simulink model "pfc_simulation"  (R2025b)
settings: Solver=ode23t  StartTime=0.0  StopTime=3  FixedStep=15.625e-6  RelTol=1e-3  EnableMultiTasking=on
PostLoadFcn:
  | mchp_pfc_foc_dsPIC33A_data
values from neighbouring files (symbols this model uses):
  R = (Vout^2)/Po    (= 96.2666666667)    [mchp_pfc_foc_dsPIC33A_data.m]
  Ts = T_pwm    (= 1.5625e-05)    [mchp_pfc_foc_dsPIC33A_data.m]
undefined symbols (not defined in the file or in its folder): Down, f_sw, Up
libraries: ee_lib x8, fl_lib x7, nesl_utility x7, eeGeneralControl x1
settings Model: ExtModeEnableFloating=off  ExtModeTrigDuration=20  Creator=I50990  LastModifiedBy=Andy
settings SolverCC: AlgebraicLoopSolver=TrustRegion
settings OptimizationCC: DefaultParameterBehavior=Inlined  DefaultUnderspecifiedDataType=single  InlineInvariantSignals=on  EnhancedBackFolding=on  BooleansAsBitfields=on  PassReuseOutputArgsAs=Individual arguments  ZeroExternalMemoryAtStartup=off  ZeroInternalMemoryAtStartup=off  OptimizeBlockOrder=speed  DifferentSizesBufferReuse=on  EfficientTunableParamExpr=on
settings DebuggingCC: MultiTaskDSMMsg=none  MultiTaskCondExecSysMsg=none  MultiTaskRateTransMsg=warning  ParameterTunabilityLossMsg=error  ArithmeticOperatorsInVariantConditions=warning
settings HardwareCC: ProdBitPerPointer=32.0  ProdBitPerSizeT=32.0  ProdBitPerPtrDiffT=32.0  ProdLargestAtomicInteger=Long  ProdWordSize=32.0  ProdLongLongMode=on  ProdHWDeviceType=Generic->Custom
settings ModelReferenceCC: ModelReferenceNumInstancesAllowed=Single
settings SFSimCC: MATLABDynamicMemAlloc=off  CustomCodeUndefinedFunction=UseInterfaceOnly
settings RTWCC: SystemTargetFile=MCHP_dsPIC33A_stf.tlc  TLCOptions="-aExtModeXCPClassicInterface=0  -aCreateExtModeTypes=1 -aExtModeXCPSimulationTimeInTicks=1"  TemplateMakefile=MCHP_dsPIC33A.tmf  GPUComputeCapability=3.5  Description=Microchip Embedded Target dsPIC33A (real-time)
settings CodeAppCC: ForceParamTrailComments=on  IgnoreCustomStorageClasses=off  MaxIdLength=255.0  OperatorAnnotations=on  SimulinkDataObjDesc=on  SFDataObjDesc=on  InsertBlockDesc=on
settings STFCustomTargetCC: SystemTargetFile=MCHP_dsPIC33A_stf.tlc  TargetLibSuffix=_lib.a  TargetLangStandard=C99 (ISO)  MultiwordLength=256.0  ConcurrentExecutionCompliant=off  CombineOutputUpdateFcns=on  CombineSignalStateStructs=on  ERTCustomFileBanners=on  SupportContinuousTime=off  RemoveResetFunc=on  MATLABClassNameForMDSCustomization=Simulink.SoftwareTarget.ERTCustomization  GRTInterface=off  TIMER_PERIOD="[0  65535]"  GCC1=xc-dsc-gcc.exe  AR1=xc-dsc-ar  OPTIM_GCC=-O2 -mno-eds-warn -mconst-in-data -mlarge-code -mlarge-data -mlarge-scalar -mlarge-aggregate -g -Wa,--reorder  GCCPATH=C:/PROGRA~1/MICROC~1/xc-dsc/v3.21/bin  AssemblyListing=off  MCHP_XCP_MemoryBlockParameters=[-1 8]  LINKER_SCRIPT=p33AK128MC106.gld  ProduceHexOutput=off  HOST_PLATFORM=PC  BIN2HEX=xc-dsc-bin2hex  TIMER_START="[0  0]"  RTWGenSettings_txt="s.UART_TX_IMPLEMENTATION='[2  2]';s.UART_RX_IMPLEMENTATION='[2  2]';s.UART_TX_DMACHANNEL='[2  1]';s.UART_HALF_DUPLEX_MODE='[0  0]';s.UART_TX_THREAD_PROTECTION='[9  9]';s.RefMasterBlk='pfc_model_simulation/MCHV-230VAC-1.5kW Development Board dsPIC33AK128MC106 MC DIM/Microchip Master';s.ChipIdN='[33  128  106]';s.ChipIdL1='AK';s.ChipIdL2='MC';s.ChipIdL3='';s.arch3='33A';s.ChipId='33AK128MC106';s.Arch='8';s.bitFieldsSFR='3';s.ChipRAM='16384';s.ChipRAM_XBegin='16384';s.ChipRAM_dma='[-1 -1]';s.FuseConfigTxt='#pragma config FWDT_WDTEN = SW\\\\n#pragma config FICD_JTAGEN = OFF\\\\n';s.TimeStep_Timer='-1';s.TimeStep_SyncADC='1';s.ADPCFG='0';s.ANSEL_Exist='1';s.ANSEL='[-1 -1 -1 -1 -1 -1 -1 -1 -1 -1 -1]';s.TRIS='[65535  65535  64990  65503     -1     -1     -1     -1     -1     -1     -1     -1     -1     -1     -1     -1     -1     -1     -1     -1     -1     -1     -1     -1     -1     -1     -1     -1     -1     -1     -1     -1     -1     -1     -1     -1     -1     -1     -1     -1     -1     -1     -1     -1     -1     -1     -1     -1     -1     -1     -1     -1     -1     -1     -1     -1     -1]';s.RPOR='[-1         -1         -1         -1         -1         -1         -1         -1         -1         -1     589824         -1         -1         -1  184549376         -1         -1         -1         -1         -1]';s.RPINR='[-1       -1       -1       -1       -1       -1       -1       -1       -1  3997740       -1       -1       -1       -1       -1       -1       -1       -1       -1       -1       -1       -1]';s.LATSET='[-1 -1 -1 -1 -1 -1 -1 -1 -1 -1 -1 -1 -1 -1 -1 -1 -1 -1 -1 -1 -1 -1 -1 -1 -1 -1 -1 -1 -1 -1 -1 -1 -1 -1 -1 -1 -1 -1 -1 -1 -1 -1 -1 -1 -1 -1 -1 -1 -1 -1 -1 -1 -1 -1 -1 -1 -1]';s.LATCLR='[-1 -1 -1 -1 -1 -1 -1 -1 -1 -1 -1 -1 -1 -1 -1 -1 -1 -1 -1 -1 -1 -1 -1 -1 -1 -1 -1 -1 -1 -1 -1 -1 -1 -1 -1 -1 -1 -1 -1 -1 -1 -1 -1 -1 -1 -1 -1 -1 -1 -1 -1 -1 -1 -1 -1 -1 -1]';s.ODC='[-1 -1 -1 -1 -1 -1 -1 -1 -1 -1 -1 -1 -1 -1 -1 -1 -1 -1 -1 -1 -1 -1 -1 -1 -1 -1 -1 -1 -1 -1 -1 -1 -1 -1 -1 -1 -1 -1 -1 -1 -1 -1 -1 -1 -1 -1 -1 -1 -1 -1 -1 -1 -1 -1 -1 -1 -1]';s.CNPU='[-1 -1 -1 -1 -1 -1 -1 -1 -1 -1 -1 -1 -1 -1 -1 -1 -1 -1 -1 -1 -1 -1 -1 -1 -1 -1 -1 -1 -1 -1 -1 -1 -1 -1 -1 -1 -1 -1 -1 -1 -1 -1 -1 -1 -1 -1 -1 -1 -1 -1 -1 -1 -1 -1 -1 -1 -1]';s.CNPD='[-1 -1 -1 -1 -1 -1 -1 -1 -1 -1 -1 -1 -1 -1 -1 -1 -1 -1 -1 -1 -1 -1 -1 -1 -1 -1 -1 -1 -1 -1 -1 -1 -1 -1 -1 -1 -1 -1 -1 -1 -1 -1 -1 -1 -1 -1 -1 -1 -1 -1 -1 -1 -1 -1 -1 -1 -1]';s.PortConfigTxt='';s.CLKDIV='0';s.PLLFBD='-1';s.PLLDIV='16815713';s.QUARTZ='8000000';s.SWITCH_OSC='16386';s.PLLRNG='-1';s.MASTER_BusyFlag='-1';s.POWERSAVE='0';s.MIPS='200000000';s.FLASH_ECC='0';s.PBxDIV='[-1]';s.CLKx_INTDIV='[-1 -1 -1 -1  0  1 -1  0  0 -1 -1  0 -1]';s.CLKx_FRACDIV='[-1   -1   -1   -1    0  256   -1    0    0   -1   -1    0   -1]';s.AN_type2='1';s.ACLKCON_reg='-1';s.nTIMERS='1';s.nSCCP='4';s.DOS_04094_cpu_33a_v1_dspic33a='1';s.DOS_04436_perseus_dspic33a='1';s.DOS_04928_gpio_ports_upb_v2_dspic33a='1';s.DOS_02672_math_progcrc_upb_v1_dspic33a='1';s.DOS_04993_sec_32bit_cp_upb_v1_dspic33a='1';s.DOS_03681_bmx_33a_upb_v1_dspic33a='0';s.DOS_03459_adc_pc_ctrl_upb_v2_dspic33a='1';s.DOS_04302_pwm_pc_upb_v3_dspic33a='1';s.DOS_03076_uart_protocol_upb_v1_dspic33a='1';s.DOS_01482_spi_i2s_upb_v1_dspic33a='1';s.DOS_05155_i2c_upb_v4_dspic33a='1';s.DOS_02359_sent_j2716_upb_v1_dspic33a='1';s.DOS_05177_qei_32b_upb_v2_dspic33a='1';s.DOS_01512_ccp_mccp_upb_v1_dspic33a='1';s.DOS_03496_dac_pdm_nbit_upb_v2_dspic33a='1';s.DOS_02673_tmr_classa_upb_v1_dspic33a='1';s.DOS_04776_perf_mon_upb_v1_dspic33a='1';s.DOS_03680_pfm_pbu_33a_upb_v1_dspic33a='1';s.DOS_04649_sec_pac_upb_v0_dspic33a='1';s.DOS_03966_io_integrity_monitor_upb_v1_dspic33a='1';s.DOS_04641_biss_master_upb_v1_dspic33a='1';s.DOS_04077_dma_upb_v1_dspic33a='1';s.DOS_04549_nvm_ctrl_32bit_upb_v1_dspic33a='1';s.DOS_04449_clk_cru_33a_upb_v1_dspic33a='1';s.DOS_03850_clk_monitor_upb_v1_dspic33a='1';s.DOS_04342_osc_rc8mhz_ctrl_upb_v4_dspic33a='1';s.DOS_04650_wdt_upb_v4_dspic33a='1';s.DOS_05178_ptg_pc_upb_v1_dspic33a='0';s.DOS_04181_data_ram_ctrl_upb_v1_dspic33a='1';s.DOS_04735_wdt_dmt_upb_v6_dspic33a='1';s.DOS_01577_cla_clc_upb_v1_dspic33a='1';s.DOS_03516_pwr_sib_upb_v3_dspic33a='1';s.DOS_03495_amp_pad_opamp_ctrl_upb_v2_dspic33a='1';s.DOS_05308_pegasus_dspic33a='0';s.DOS_02976_adc_12b_upb_v2_dspic33a='0';s.DOS_05404_adc_pc_ctrl_upb_v3_dspic33a='0';s.DOS_05226_pwm_pc_upb_v4_dspic33a='0';s.DOS_05226_apwm_pc_upb_v4_dspic33a='0';s.DOS_05431_dac_pdm_nbit_upb_v3_dspic33a='0';s.DOS_04649_sec_pac_upb_v1_dspic33a='0';s.DOS_05461_pwr_sib_upb_v4_dspic33a='0';s.DOS_05420_amp_vref_ctl_upb_v1_dspic33a='0';s.DOS_03267_adc_soft_code_seq_v1_dspic33a='0';s.DOS_04537_can_fd_upb_v3_dspic33a='0';s.DOS_05346_sec_cam_lite_v2_dspic33a='0';s.DOS_05830_blueRidge_dspic33a='0';s.DOS_05972_adc_12b_upb_v3_itc_dspic33a='0';s.DOS_05514_qei_32b_upb_v3_dspic33a='0';s.DOS_05765_math_rdc_upb_v1_32bit='0';s.DOS_05908_math_cic_upb_v2_32bit='0';s.DOS_05801_dma_upb_v2_dspic33a='0';s.DOS_05592_pwr_monitor_sib_upb_v1='0';s.DOS_05924_bus_dual_die_upb_v2='0';s.DOS_05922_i3c_upb_v1_32bit='0';s.DOS_06006_adc_soft_code_seq_v2_dspic33a='0';s.DOS_05442_icd_trace_33a_v1_dspic33a='0';s.DOS_02551_cpu_16bit_v7='0';s.DOS_01520_wdt_dmt_upb_v1_16bit='0';s.DOS_02359a_sent_j2716_upb_v1='0';s.DOS_02672_math_progcrc_upb_v1_16bit='0';s.DOS_01577_cla_clc_upb_v1='0';s.DOS_02915_ecc_v2='0';s.DOS_02673_tmr_classa_upb_v1_16bit='0';s.DOS_01494_qei_32b_upb_v1_16bit='0';s.DOS_02472_ppi_pmp16_upb_v1_16bit='0';s.DOS_01441_i2c_upb_v1_16bit_TLAH='0';s.DOS_03076_uart_protocol_upb_v1_16bit='0';s.DOS_01482='0';s.DOS_01483_pwm_16bit='0';s.DOS_02949_WACG='0';s.DOS_02316_nvm_ctrl_v1_16bit='0';s.DOS_03349_amp_pad_opamp_ctrl_upb_v1='0';s.DOS_02653_afe_current_bias_ctrl_upb_v1_16bit='0';s.DOS_01459_ptg_pc_upb_v1_16bit='0';s.DOS_01512_ccp_mccp_upb_v1_16bit='0';s.DOS_02519_dma_sfr_16bit_v2='0';s.DOS_02508c11='0';s.DOS_02475_dac_pdm_nbit_upb_v1_16bit='0';s.DOS_02467_gpio_upb_v1_16bit='0';s.DOS_00805_rst_integration_v4='0';s.DOS_02659_clk_sib_v12='0';s.DOS_02237_osc_dco_ctrl_upb_v1_16bit='0';s.DOS_02674_wdt_upb_v1_16bit='0';s.DOS_01407='0';s.DOS_03247_CAN_FD_UPB_V2_16_bit='0';s.DOS_03994_WAC07='0';s.DOS_02552_msi_upb_v1_Master='0';s.DOS_03667_pwm_pc_upb_v2_16bit='0';s.DOS_04180_drm_ctrl_ecc_v1='0';s.DOS_03431_STX03='0';s.DOS_03516_pwr_sib_upb_v3='0';s.DOS_02552_msi_upb_v1_Slave='0';s.DOS_04621_amp_pga_ctrl_upb_v3='0';s.DOS_02497_WACV='0';s.DOS_02593_amp_pga_ctrl_pb_v2_16bit='0';s.DOS_01461_afe_ctmu_con_upb_v1_16bit='0';s.DOS_02497_WACA='0';s.DOS_02478_uart_irda_upb_v1_16bit='0';s.DOS_00929='0';s.DOS_01198='0';s.DOS_03029_WACH='0';s.DOS_01483_apwm_16bit='0';s.DOS_04797_WAC0A='0';s.DOS_04884_WAC0B='0';s.DOS_04797_WAC09='0';s.DOS_03662_WACU='0';s.DOS_00794='0';s.DOS_00931='0';s.DOS_00932='0';s.DOS_00942='0';s.DOS_00938='0';s.DOS_00996='0';s.DOS_00997='0';s.DOS_00998='0';s.DOS_00209='0';s.DOS_01555_adc='0';s.DOS_01293='0';s.DOS_00828='0';s.DOS_01116='0';s.DOS_01017_RPORx='0';s.DOS_01017_RPINRx='0';s.DOS_01555_nvm_tsmc18_v2_16bit='0';s.DOS_00804='0';s.DOS_00826='0';s.DOS_01555_TLAK_PMDx='0';s.DOS_01555_TLAK_INT_='0';s.DOS_00933='0';s.DOS_01555='0';s.DOS_01555_ptg='0';s.DOS_00958='0';s.DOS_01117_PORTx='0';s.DOS_00999='0';s.DOS_01041='0';s.DOS_00892='0';s.DOS_01287_TLAC_PMDx='0';s.DOS_01287_TLAC_INT_='0';s.DOS_01424='0';s.DOS_01332='0';s.DOS_01468_PMBA_current_source='0';s.DOS_02291_PGA='0';s.DOS_01467_Comparator='0';s.DOS_01498_TLAY='0';s.DOS_00993_PLL_120MHz='0';s.DOS_01332_ptg_pc_v1='0';s.DOS_00958_pwm_TLAY='0';s.TLAY_IOPorts='0';s.DOS_00929q='0';s.DOS_02415_spi_v5='0';s.DOS_RPINRx_16bit_2='0';s.DOS_01497_TLAH_PMDx='0';s.DOS_02550_TLAL_INT='0';s.DOS_00958_pwm_TLAH='0';s.DOS_01287_TLAH_INT_='0';s.DOS_01113='0';s.DOS_01017_PMDx='0';s.DOS_00927='0';s.DOS_01080='0';s.DOS_00794_cpu_16bit_v3='0';s.DOS_02192_TLCD_PMDx='0';s.DOS_02192_TLCD_INT_='0';s.DOS_02192_cmp='0';s.DOS_00958_pwm_TLCD='0';s.DOS_02192_PORTx_TLCD='0';s.DOS_00936='0';s.DOS_00995='0';s.DOS_00546='0';s.DOS_00474='0';s.DOS_02481_WACK_MC_Config='0';s.DOS_03088_pfm_cache_ocp_v2_WACK='0';s.DOS_02819_pfm_ctrl_32bit_upb_v2='0';s.DOS_02674_wdt_upb_v1_32bit='0';s.DOS_01520_wdt_dmt_upb_v1='0';s.DOS_02869_icd_jtag_bvci_upb_v2='0';s.DOS_02823_WACJ_clk_cru_upb_v2='0';s.DOS_02823_WACN_clk_cru_upb_v2='0';s.DOS_01423_RPINRx='0';s.DOS_02481_RPORx='0';s.DOS_02511_pwr_sib_upb_v1_32bit='0';s.DOS_02907_WACN_GP_int_evic_v3='0';s.DOS_01500_dma_bvci_v2='0';s.DOS_02141_tmr_classa_pb_v2='0';s.DOS_02815_tmr_classb_upb_v1='0';s.DOS_00740_icap_pb_v1='0';s.DOS_00749_ocmp_pb_v1='0';s.DOS_01441_i2c_upb_v1_32bit='0';s.DOS_01329_spi_pb_v2='0';s.DOS_02478_uart_irda_upb_v1_32bit='0';s.DOS_03554_cmp_control_upb_v2_32bit='0';s.DOS_01445_dac_nbit__control_upb_v1_32bit='0';s.DOS_01461_afe_ctmu_con_upb_v1='0';s.DOS_01577_cla_clc_upb_v1_32bit='0';s.DOS_02467_gpio_ports_upb_v1='0';s.DOS_02508_adc_sar_ctrl_upb_v1_PIC32MK='0';s.DOS_01261_tmr_rtcc_pb_v2='0';s.DOS_01475_lpwr_deep_sleep_ctrl_v2='0';s.DOS_EIP_00136_ssx_v1='0';s.DOS_02907_WACN_MC_int_evic_v3='0';s.DOS_01477_pwm_mc_upb_v1='0';s.DOS_01494_qei_32b_upb_v1='0';s.DOS_03247_can_fd_upb_v2_pic32mk='0';s.DOS_02907_WACK_MC_int_evic_v3='0';s.DOS_02514_dfm_strl_sst_upb_v1='0';s.DOS_02472_ppi_pmp16_upb_v1='0';s.DOS_02813a_usb_otgcore_pb_v3='0';s.DOS_02481_WACJ_MC_Config='0';s.DOS_02569_pfm_cache_ocp_v1='0';s.DOS_02481_WACJ_MC_int_evic_v3='0';s.DOS_01459_ptg_pc_upb_v1_SIC='0';s.DOS_01427_cmp_control_upb_v1_32bit='0';s.DOS_01152_can_bvci_v1='0';s.DOS_02787_WACD_Config='0';s.DOS_00800_dac_4bit_ctrl_pb_v1='0';s.DOS_01539_icd_jtag_pb_v2='0';s.DOS_02823_clk_cru_upb_v2='0';s.DOS_01423_RPORx='0';s.DOS_02907_WACD_int_evic_v3='0';s.DOS_00734_uart_irda_pb_v1='0';s.DOS_00687_tmr_classa_pb_v1='0';s.DOS_00745_tmr_classb_pb_v1='0';s.DOS_02508_adc_sar_ctrl_upb_v1='0';s.DOS_00866_cmp_control_pb_v2='0';s.DOS_01114_eth_bvci_v1='0';s.DOS_02831_usb_clk_rst_v2='0';s.DOS_01643_pfm_cache_ahb_v2='0';s.DOS_EIP_00206r5_sqi_v2='0';s.DOS_EIP_00124_usb_hs_otgcore_v1='0';s.DOS_EIP_00218_math_rng_ahbs_v2='0';s.DOS_EIP_00109_ebi_v1='0';s.DOS_EIP_00158_crypto_v1='0';s.DOS_05178_ptg_pc_upb_v2_dspic33a='1';s.DOS_05346_sec_cam_v2_dspic33a='0';s.DOS_05557_serpens_dspic33a='0';s.DOS_05972_adc_12b_upb_v3_adc_dspic33a='0';s.DOS_02050_tmr_rtcc_upb_v1_dspic33a='0';s.DOS_04649_sec_pac_upb_serpens_dspic33a='0';s.DOS_05692_pwr_sib_upb_v5_dspic33a='0';s.DOS_06006_adc_soft_code_seq_v2_adc_dspic33a='0';s.DOS_02481_WACP_Config='0';s.DOS_02907_WACP_int_evic_v3='0';s.DOS_02508_WACP_adc_sar_ctrl_upb_v1='0';s.DOS_01261_tmr_rtcc_WACJ_K_N_P_pb_v2='0';"  MCHP_AUTO_FLASH=off  PIC_REF=33AK128MC106  TIMER_PRESCALER="[-1  0 -1 -1 -1]"  LDFLAGS='--report-mem,-Map=$(PRODUCT_NAME).map,-cref,-lq-dsp,--memorysummary,memoryfile.xml'  MCHP_CompiledTime_ModelSampleTimes_Txt=s(1).Value=reshape([1.5625e-05 0],1,2);s(1).Description='Discrete 1';s(1).ColorRGBValue=reshape(MCHP_Fun.Hex2num('[3FF0000000000000 3FD1515151515151 3FCD1D1D1D1D1D1D]'),1,3);s(1).Annotation='D1';s(1).TID=0;s(1).Owner=[];s(1).ComponentSampleTimes=[];s(2).Value=reshape([0.00015625 0],1,2);s(2).Description='Discrete 2';s(2).ColorRGBValue=reshape(MCHP_Fun.Hex2num('[3FCD1D1D1D1D1D1D 3FE9191919191919 3FC8989898989899]'),1,3);s(2).Annotation='D2';s(2).TID=1;s(2).Owner=[];s(2).ComponentSampleTimes=[];s(3).Value=reshape([0.0005 0],1,2);s(3).Description='Discrete 3';s(3).ColorRGBValue=reshape(MCHP_Fun.Hex2num('[3FAC1C1C1C1C1C1C 0000000000000000 3FF0000000000000]'),1,3);s(3).Annotation='D3';s(3).TID=2;s(3).Owner=[];s(3).ComponentSampleTimes=[];s(4).Value=reshape([0.02 0],1,2);s(4).Description='Discrete 4';s(4).ColorRGBValue=reshape(MCHP_Fun.Hex2num('[3FAC1C1C1C1C1C1C 0000000000000000 3FF0000000000000]'),1,3);s(4).Annotation='D4';s(4).TID=3;s(4).Owner=[];s(4).ComponentSampleTimes=[];s(5).Value=reshape([0.1 0],1,2);s(5).Description='Discrete 5';s(5).ColorRGBValue=reshape(MCHP_Fun.Hex2num('[3FAC1C1C1C1C1C1C 0000000000000000 3FF0000000000000]'),1,3);s(5).Annotation='D5';s(5).TID=4;s(5).Owner=[];s(5).ComponentSampleTimes=[];s(6).Value=reshape([0.5 0],1,2);s(6).Description='Discrete 6';s(6).ColorRGBValue=reshape(MCHP_Fun.Hex2num('[3FAC1C1C1C1C1C1C 0000000000000000 3FF0000000000000]'),1,3);s(6).Annotation='D6';s(6).TID=5;s(6).Owner=[];s(6).ComponentSampleTimes=[];s(7).Value=reshape([Inf Inf],1,2);s(7).Description='Constant';s(7).ColorRGBValue=reshape(MCHP_Fun.Hex2num('[3FEA3A3A3A3A3A3A 3F90101010101010 3FE1717171717171]'),1,3);s(7).Annotation='Inf';s(7).TID=-2;s(7).Owner=[];s(7).ComponentSampleTimes=[];s(8).Value='Source: D5';s(8).Description='Triggered';s(8).ColorRGBValue=reshape(MCHP_Fun.Hex2num('[3FAC1C1C1C1C1C1C 0000000000000000 3FF0000000000000]'),1,3);s(8).Annotation='D5';s(8).TID=8;s(8).Owner=[];s(8).ComponentSampleTimes=[];s(9).Value=[];s(9).Description='Multirate';s(9).ColorRGBValue=reshape(MCHP_Fun.Hex2num('[3FE1717171717171 3FD999999999999A 3F98181818181818]'),1,3);s(9).Annotation='M';s(9).TID=[];s(9).Owner=[];s(9).ComponentSampleTimes=[];  EXTMODE_DATA_UPLOAD=on  OBJDUMP=xc-dsc-objdump  MCHP_MULTITHREAD_COMPILATION=on  LinkWithMaster=off
settings ERTTargetCC: ExtModeTransport=1.0  ExtModeStaticAlloc=on  ExtModeStaticAllocSize=2048.0  ExtModeMexFile=ext_xcp  ExtModeIntrfLevel=Level2 - Open  ERTSrcFileBannerTemplate=MCHP_dsPIC_code_template.cgt  ERTHdrFileBannerTemplate=MCHP_dsPIC_code_template.cgt  ERTDataSrcFileTemplate=MCHP_dsPIC_code_template.cgt  ERTDataHdrFileTemplate=MCHP_dsPIC_code_template.cgt  ERTCustomFileTemplate=MCHP_main.tlc  MaxLineWidth=110.0  DynamicArrayContainerType=coder::array  TargetLibSuffix=_lib.a  TargetLangStandard=C99 (ISO)  ParMdlRefBuildCompliant=off  CompOptLevelCompliant=off  ConcurrentExecutionCompliant=off  CombineSignalStateStructs=on  SupportNonInlinedSFcns=on  ModelStepFunctionPrototypeControlCompliant=off  CPPClassGenCompliant=off  UseToolchainInfoCompliant=off

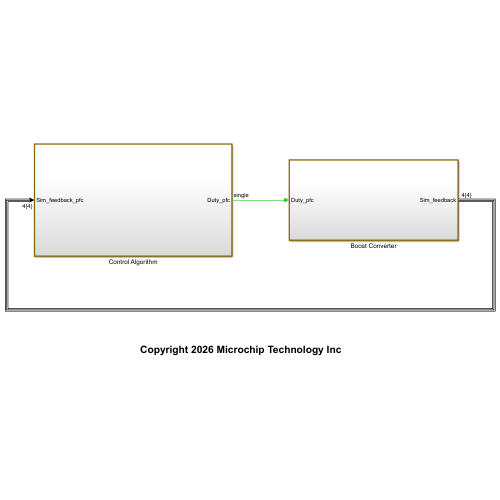
[thumbnail: Simulink's stored preview of the top-level diagram]
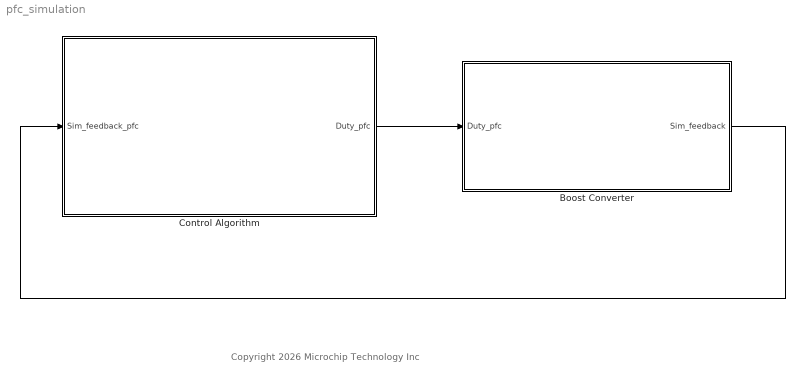
== system pfc_simulation ==
  note: Copyright 2026 Microchip Technology Inc
  Boost Converter : Subsystem
  Control Algorithm : Subsystem
  wires:
  Control Algorithm/1(Duty_pfc) -> Boost Converter/1(Duty_pfc)
  Boost Converter/1(Sim_feedback) -> Control Algorithm/1(Sim_feedback_pfc)

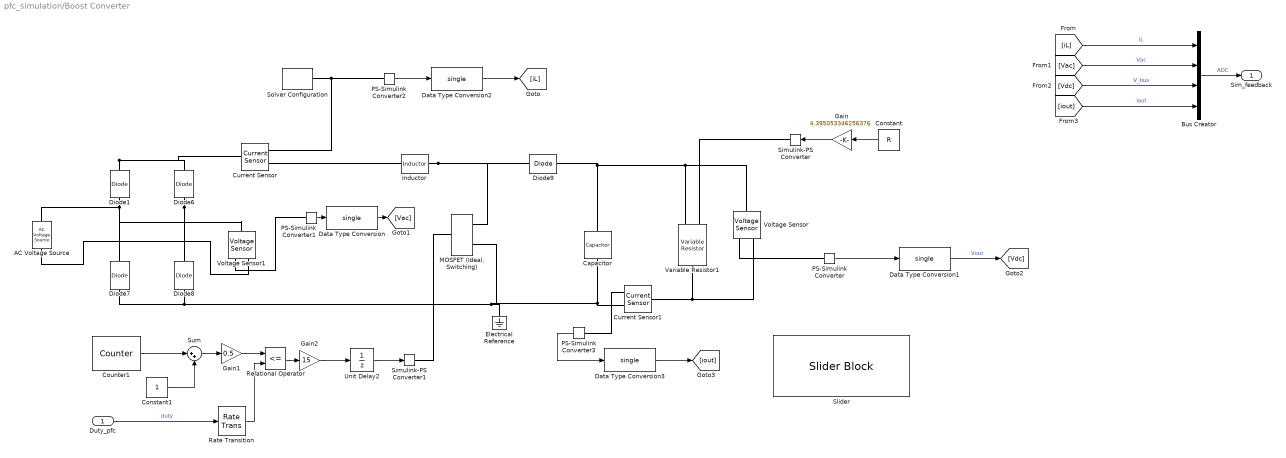
== system pfc_simulation/Boost Converter ==
  Duty_pfc : Inport
  AC Voltage Source : fl_lib/Electrical/Electrical Sources/AC Voltage Source  amp=230 V  shift=0 deg  frequency=50 Hz
  Bus Creator : BusCreator  Inputs=4
  Capacitor : ee_lib/Passive/Capacitor  cap_option=ee.enum.passive.capacitor.capOption.const  c=C F  Cvec=[1e-05, 1e-06] F  Vvec=[0, 10] V  CV_table_symmetry=ee.enum.passive.capacitor.tableSymmetry.yes  f_vec=[1, 10] kHz  DFext_vec=[.8, 1.2]  enable_C_tol=ee.enum.toleranceApplication.none  averaging_period=0 s  C_tol=5  tol_distribution=ee.enum.toleranceDistribution.uniform  nSigma=4  r=0 Ohm  g=0 1/Ohm  enable_operating_limits=ee.enum.enable.no  operating_limit_action=ee.enum.passive.reportOpLim.warn  max_working_voltage_range=[-25, 25] V  power_rating=1 W  maxTemperature=85 degC  thermalEnable=false  thermalMass=1 J/K  i_specify=off  i_priority=None  i=0 A  i_nominal_specify=off  i_nominal_value=1  i_nominal_unit=A  v_specify=off  v_priority=None  v=0 V  v_nominal_specify=off  v_nominal_value=1  v_nominal_unit=V  vc_specify=off  vc_priority=High  vc=0 V  vc_nominal_specify=off  vc_nominal_value=1  vc_nominal_unit=V  T_specify=off  T_priority=None  T=298.15 K  T_nominal_specify=off  T_nominal_value=1  T_nominal_unit=K
  Constant : Constant  Value=R  SampleTime=Ts
  Constant1 : Constant  SampleTime=Ts
  Counter1 : eeGeneralControl/Counter  CarrCount=Up-Down  Range=[-1 1]  Tper=Ts/2  Tdelay=Ts/2  Ts=Ts/40
  Current Sensor : fl_lib/Electrical/Electrical Sensors/Current Sensor
  Current Sensor1 : fl_lib/Electrical/Electrical Sensors/Current Sensor
  Data Type Conversion{,1..3} (4 alike) : DataTypeConversion  OutDataTypeStr=single  ConvertRealWorld=Stored Integer (SI)  SaturateOnIntegerOverflow=off  RndMeth=Floor
  Diode{1,6..9} (5 alike) : ee_lib/Semiconductors & Converters/Diode  ModelType=ee.enum.diode.modelType.pwl  TableType=ee.enum.diode.tableType.IfMat  IfMat=[.07, .12, .19, 1.75, 4.24, 7.32, 11.2; .16, .3, .72, 2.14, 5.02, 8.35, 13.12] A  VfMat=[.9, 1.15, 1.25, 1.5, 1.75, 2.17, 2.6, 2.85; .58, .68, .75, 1.1, 1.38, 1.77, 2.27, 2.7] V  TjVec=[25, 125] degC  VfVec=[.5, .7, .9, 1.3, 1.7, 2.1, 2.5] V  IfVec=[.1, .2, .5, 1, 2, 4, 7, 10] A  IrMat=[1e-06, 2e-06, 5e-06, 1e-05, 2.5e-05, 5e-05, .0001; 2e-06, 5e-06, 1e-05, 4e-05, 8e-05, .0002, .0005] A  VrMat=[10, 100, 200, 250, 300, 325, 350; 10, 70, 160, 220, 270, 300, 320] V  VrVec=[10, 20, 40, 50, 70, 80, 100] V  IrVec=[1e-06, 2e-06, 5e-06, 1e-05, 2e-05, 5e-05, .0001] A  Vf=0.6 V  Ron=0.3 Ohm  Goff=1e-8 S  prmExp=ee.enum.diode.expParam.useTwo  I12=[.0137, .545] A  V12=[.6, .7] V  RS=0 Ohm  Tmeas=298.15 K  IS=1e-12 A  ec=1  I1=0.0137 A  V1=0.6 V  N_series=1  N_parallel=1  ZenerEnable=false  Rz=0.3 Ohm  BV=inf V  C_param=ee.enum.diode.capParam.fixed  CJ=0 pF  CJ0=5 pF  Vvec=[.1, 10, 100] V  Cvec=[3.5, 1, .4] pF  VJ=1 V  Mgrad=0.5  FC=0.5  Q_param=ee.enum.diode.recoveryParam.off  iRM=-7.15 A  iF=4 A  didt=-750 A/us  trr_factor=3  trr=115 ns  Qrr=150 nA*s  Vr=-600 V  Ls=150 nH  Erec=0.03 J  TT=50 ns  tau=100 ns  T_param=ee.enum.diode.temperatureParam.off  Tdevice=298.15 K  I1_T2=0.245 A  V1_T2=0.5 V  IS_T2=1.25e-7 A  Tmeas2=125 degC  XTI_param=ee.enum.diode.xtiParam.pn  XTI=3  EG_param=ee.enum.diode.egapParam.material_si  EG=1.11 eV  dBVdT=0 V/K  enable_fault_input=simscape.enum.onoff.off  i_specify=off  i_priority=None  i=0 A  i_nominal_specify=off  i_nominal_value=1  i_nominal_unit=A  v_specify=off  v_priority=None  v=0 V  v_nominal_specify=off  v_nominal_value=1  v_nominal_unit=V  v_capacitor_specify=off  v_capacitor_priority=None  v_capacitor=0 V  v_capacitor_nominal_specify=off  v_capacitor_nominal_value=1  v_capacitor_nominal_unit=V  Qj_specify=off  Qj_priority=High  Qj=0 C  Qj_nominal_specify=off  Qj_nominal_value=1  Qj_nominal_unit=C  i_diode_specify=off  i_diode_priority=None  i_diode=0 A  i_diode_nominal_specify=off  i_diode_nominal_value=1  i_diode_nominal_unit=A  v_diode_specify=off  v_diode_priority=None  v_diode=0 V  v_diode_nominal_specify=off  v_diode_nominal_value=1  v_diode_nominal_unit=V  i_capacitor_specify=off  i_capacitor_priority=None  i_capacitor=0 A  i_capacitor_nominal_specify=off  i_capacitor_nominal_value=1  i_capacitor_nominal_unit=A  power_dissipated_specify=off  power_dissipated_priority=None  power_dissipated=0 W  power_dissipated_nominal_specify=off  power_dissipated_nominal_value=1  power_dissipated_nominal_unit=W  fidelity_level=ee.enum.diode.fidelity.includeChargeDyn  rec_loss_model=ee.enum.diode.reverseRecoveryModel.fixed  ErecVal=0 J  scaleWithIandV=true  ErecMat=zeros(2, 3) J  TjrecVec=[298.15, 398.15] K  IfrecVec=[.1, 1, 10] A  IrecVal=10 A  VrecVal=10 V  tFilter=1 / 1000 / 100 s  thermal_network_parameterization=ee.enum.thermalNetworkTopology.junctionCase  Rth=[0, 10] K/W  Rth_Cauer=[1, 3, 10] K/W  Rth_Foster=[.08, .14, .22, .16] K/W  thermal_mass_parameterization=ee.enum.thermalNetwork.timeconstant  thermal_mass=[0, 1] J/K  thermal_mass_Cauer=[.1, .3, 1] J/K  thermal_mass_Foster=[.001, .005, .05, .5] J/K  thermal_time_constant=[0, 10] s  thermal_time_constant_Cauer=[1, 3, 10] s  thermal_time_constant_Foster=[7e-05, .0007, .01, .08] s  thermal_mass_initial_temperatures=[25, 25] degC  thermal_mass_initial_temperatures_Cauer=[25, 25, 25] degC  junction_thermal_mass=0.01 J/K  Tvec_initial_Foster=[25, 25, 25, 25] degC  no_thermal_network=0  junction_temperature_specify=off  junction_temperature_priority=None  junction_temperature=25 degC  junction_temperature_nominal_specify=off  junction_temperature_nominal_value=1  junction_temperature_nominal_unit=degC
  Electrical Reference : fl_lib/Electrical/Electrical Elements/Electrical Reference
  Gain : Gain  Gain=4.395053346256376
  Gain1 : Gain  Gain=0.5
  Gain2 : Gain  Gain=15  OutDataTypeStr=double
  Inductor : ee_lib/Passive/Inductor  l=L H  enable_L_tol=ee.enum.toleranceApplication.none  L_tol=20  tol_distribution=ee.enum.toleranceDistribution.uniform  nSigma=4  r=0 Ohm  g=1e-9 1/Ohm  enable_operating_limits=ee.enum.enable.no  operating_limit_action=ee.enum.passive.reportOpLim.warn  max_working_current=1 A  power_rating=1 W  i_L_specify=off  i_L_priority=High  i_L=0 A  i_L_nominal_specify=off  i_L_nominal_value=1  i_L_nominal_unit=A
  "MOSFET (Ideal, Switching)" : ee_lib/Semiconductors & Converters/MOSFET (Ideal, Switching)  port_option=ee.enum.controlport.ps  Rds=0.01 Ohm  Goff=1e-6 1/Ohm  Vth=2 V  diode_param=ee.enum.semiconductors.protectionDiode.nodynamics  diode_Vf=0.8 V  diode_Ron=0.001 Ohm  diode_Goff=1e-5 1/Ohm  diode_C=50e-9 F  diode_iRM=-235 A  diode_iF=300 A  diode_idot=-50 A/us  diode_trr_param=ee.enum.converters.diodeReverseParam.trr_factor  diode_trr_factor=3  diode_trr=15 us  diode_Qrr=1500 s*uA  ids_specify=off  ids_priority=None  ids=0 A  ids_nominal_specify=off  ids_nominal_value=1  ids_nominal_unit=A  vds_specify=off  vds_priority=None  vds=0 V  vds_nominal_specify=off  vds_nominal_value=1  vds_nominal_unit=V  vgs_specify=off  vgs_priority=None  vgs=0 V  vgs_nominal_specify=off  vgs_nominal_value=1  vgs_nominal_unit=V  thermal_loss_option=ee.enum.converters.thermalLossOption.constantvalues  Von_data=[0, 1.8, 3.2, 6, 10, 16; 0, 2, 5.5, 9.5, 15, 25] V  Tj=[298.15, 448.15] K  Iout_data=[0, 20, 40, 60, 80, 100] A  Eon_data=[0, 55.04, 124.57, 235.53, 362.12; 0, 71.25, 161.25, 304.88, 468.75] * 1e-6 J  Eoff_data=[0, 18, 30, 56.1, 76.5; 0, 22.5, 37.5, 70.13, 95.63] * 1e-6 J  Eon_data_3D=[zeros(2, 5, 3)] J  Eoff_data_3D=[zeros(2, 5, 3)] J  Tj_loss=[298.15, 448.15] K  Iout_data_loss=[0, 10, 20, 30, 40] A  tabulateWithVds=false  Vds_loss=[0, 150, 300] V  Eon_scalar=22.86e-3 J  Eoff_scalar=17.14e-3 J  Voff=300 V  Iout_scalar=600 A  useCurrentFromPreviousCycle=false  useVoltageFromPreviousCycle=false  diodeModelType=ee.enum.converters.diodeModelType.pwl  diodeTableType=ee.enum.diode.tableType.IfMat  diode_ReverseIVType=ee.enum.diode.diodeReverseIV.constant  diode_IfMat=[.07, .12, .19, 1.75, 4.24, 7.32, 11.2; .16, .3, .72, 2.14, 4.02, 6.35, 9.12] A  diode_VfMat=[.9, 1.15, 1.25, 1.5, 1.75, 2.17, 2.6, 2.85; .58, .68, .75, 1.1, 1.38, 1.77, 2.27, 2.7] V  diode_TjVec=[25, 125] degC  diode_VfVec=[.5, .7, .9, 1.3, 1.7, 2.1, 2.5] V  diode_IfVec=[.1, .2, .5, 1, 2, 4, 7, 10] A  diode_IrMat=[1e-06, 2e-06, 5e-06, 1e-05, 2.5e-05, 5e-05, .0001; 2e-06, 5e-06, 1e-05, 4e-05, 8e-05, .0002, .0005] A  diode_VrMat=[10, 100, 200, 250, 300, 325, 350; 10, 70, 160, 220, 270, 300, 320] V  diode_VrVec=[10, 20, 40, 50, 70, 80, 100] V  diode_IrVec=[1e-06, 2e-06, 5e-06, 1e-05, 2e-05, 5e-05, .0001] A  diode_Vr=-600 V  diode_Ls=150 nH  diode_Erec=0.03 J  diode_rec_loss_model=ee.enum.diode.reverseRecoveryModel.fixed  diode_ErecVal=0 J  diode_scaleWithIandV=true  diode_ErecMat=zeros(2, 3) J  diode_TjrecVec=[298.15, 398.15] K  diode_IfrecVec=[.1, 1, 10] A  diode_IrecVal=10 A  diode_VrecVal=10 V  diode_tFilter=1 / 1000 / 100 s  separateThermalPortForDiode=false  thermal_network_parameterization=ee.enum.thermalNetworkTopology.external  Rth=[.03, .2] K/W  Rth_Cauer=[.03, .1, .2] K/W  Rth_Foster=[.08, .14, .22, .16] K/W  thermal_mass_parameterization=ee.enum.thermalNetwork.timeconstant  thermal_mass=[3, 25] J/K  thermal_mass_Cauer=[3, 10, 25] J/K  thermal_mass_Foster=[.001, .005, .05, .5] J/K  thermal_time_constant=[.1, 5] s  thermal_time_constant_Cauer=[.1, 1, 5] s  thermal_time_constant_Foster=[7e-05, .0007, .01, .08] s  thermal_mass_initial_temperatures=[25, 25] degC  thermal_mass_initial_temperatures_Cauer=[25, 25, 25] degC  junction_thermal_mass=0.1 J/K  Tvec_initial_Foster=[25, 25, 25, 25] degC  RthDiode=[.03, .2] K/W  RthCauerDiode=[.03, .1, .2] K/W  RthFosterDiode=[.03, .2] K/W  thermalMassDiode=[3, 25] J/K  thermalMassCauerDiode=[3, 10, 25] J/K  thermalMassFosterDiode=[33, 50] J/K  thermalTauDiode=[.1, 5] s  thermalTauCauerDiode=[.1, 1, 5] s  thermalTauFosterDiode=[1, 10] s  thermalMassInitTempDiode=[25, 25] degC  thermalMassInitTempCauerDiode=[25, 25, 25] degC  junctionthermalMassDiode=0.1 J/K  TVecInitialFosterDiode=[25, 25, 25, 25] degC  no_thermal_network=0  mosfet_junction_temperature_specify=off  mosfet_junction_temperature_priority=None  mosfet_junction_temperature=25 degC  mosfet_junction_temperature_nominal_specify=off  mosfet_junction_temperature_nominal_value=1  mosfet_junction_temperature_nominal_unit=degC  diode_junction_temperature_specify=off  diode_junction_temperature_priority=None  diode_junction_temperature=25 degC  diode_junction_temperature_nominal_specify=off  diode_junction_temperature_nominal_value=1  diode_junction_temperature_nominal_unit=degC  Qj_specify=off  Qj_priority=None  Qj=0 W  Qj_nominal_specify=off  Qj_nominal_value=1  Qj_nominal_unit=W  accumulatedSwitchingLosses_specify=off  accumulatedSwitchingLosses_priority=None  accumulatedSwitchingLosses=0 J
  PS-Simulink Converter{,1..3} (4 alike) : nesl_utility/PS-Simulink Converter  PhysicalDomain=network_engine_domain  SubClassName=ps_output  LeftPortType=input  RightPortType=output  PseudoPeriodic=off  Frequencies=[]  VectorFormat=inherit  Unit=inherit  AffineConversion=off
  Rate Transition : RateTransition
  Relational Operator : RelationalOperator  Operator=<=  OutDataTypeStr=boolean  RndMeth=Simplest  InputSameDT=off
  Simulink-PS Converter : nesl_utility/Simulink-PS Converter  PhysicalDomain=network_engine_domain  SubClassName=ps_input  LeftPortType=input  RightPortType=output  PseudoPeriodic=off  Frequencies=[]  NoiseDistribution=none  NoiseParameters=[]  Unit=1  AffineConversion=off  FilteringAndDerivatives=provide  SimscapeFilterOrder=1  InputFilterTimeConstant=0.001  UdotUserProvided=0
  Simulink-PS Converter1 : nesl_utility/Simulink-PS Converter  PhysicalDomain=network_engine_domain  SubClassName=ps_input  LeftPortType=input  RightPortType=output  PseudoPeriodic=off  Frequencies=[]  NoiseDistribution=none  NoiseParameters=[]  Unit=1  AffineConversion=off  FilteringAndDerivatives=provide  SimscapeFilterOrder=1  InputFilterTimeConstant=0.001  UdotUserProvided=0
  Slider : SliderBlock  ScaleMin=1  ScaleMax=5
  Solver Configuration : nesl_utility/Solver Configuration  PhysicalDomain=network_engine_domain  SubClassName=solver  LeftPortType=input  RightPortType=generic  Tones=[]  Harmonics=[]  SimulateNoise=off  Profile=off  UseLocalSampling=off  EnableSwitchedLinearOptims=on  FrequencyDomain=off  UseCCode=off  RelTol=0.001  AbsTol=0.001  MinStep=1e-09  ToWorkspace=off  RevertToSquareIcSolve=off  NumHomotopyIterations=100  PhasorMode=off  PhasorModeNumHarmonics=1  ConsistencySolver=NEWTON_XTOL_AFTER_FTOL  IndexReductionMethod=DerivativeReplacement  DoDC=off  ResidualTolerance=1e-09  ConsistencyTolSource=GLOBAL  ConsistencyAbsTol=0.001  ConsistencyRelTol=0.001  ConsistencyTolFactor=0.001  UseLocalSolver=off  LocalSolverChoice=NE_BACKWARD_EULER_ADVANCER  ResolveIndetEquations=on  FunctionEvalNumThread=1  LocalSolverSampleTime=0.001  DoFixedCost=off  MaxNonlinIter=3  MaxModeIter=2  ComputeImpulses=off  ImpulseIterations=2  LinearAlgebra=auto  LinearAlgebraNumThread=0  EquationFormulation=NE_TIME_EF  DelaysMemoryBudget=1024  AutomaticFiltering=on  FilteringTimeConstant=0.001  PartitionStorageMethod=AS_NEEDED  PartitionMemoryBudget=1024  PartitionMethod=ROBUST  MultibodyUseLocalSolver=off  MultibodyLocalSolverChoice=ODE1  MultibodyLocalSolverSampleTime=0.001
  Sum : Sum  Inputs=|++
  Unit Delay2 : UnitDelay  SampleTime=-1  HasFrameUpgradeWarning=on
  Variable Resistor1 : fl_lib/Electrical/Electrical Elements/Variable Resistor  Rmin=R Ohm  thermalEnable=false  thermal_mass=1 J/K  i_specify=off  i_priority=None  i=0 A  i_nominal_specify=off  i_nominal_value=1  i_nominal_unit=A  v_specify=off  v_priority=None  v=0 V  v_nominal_specify=off  v_nominal_value=1  v_nominal_unit=V  T_specify=off  T_priority=None  T=300 K  T_nominal_specify=off  T_nominal_value=1  T_nominal_unit=K
  Voltage Sensor : fl_lib/Electrical/Electrical Sensors/Voltage Sensor
  Voltage Sensor1 : fl_lib/Electrical/Electrical Sensors/Voltage Sensor
  Sim_feedback : Outport
  wires:
  Gain/1 -> Simulink-PS Converter/1
  PS-Simulink Converter1/1 -> Data Type Conversion/1
  Counter1/1 -> Sum/1
  [Vac] -> Bus Creator/2  "Vac"
  Constant1/1 -> Sum/2
  Data Type Conversion1/1 -> [Vdc]  "Vout"
  [Vdc] -> Bus Creator/3  "V_bus"
  [iL] -> Bus Creator/1  "iL"
  Sum/1 -> Gain1/1
  Constant/1 -> Gain/1
  PS-Simulink Converter2/1 -> Data Type Conversion2/1
  Gain1/1 -> Relational Operator/1
  PS-Simulink Converter/1 -> Data Type Conversion1/1
  Relational Operator/1 -> Gain2/1
  Data Type Conversion/1 -> [Vac]
  Data Type Conversion2/1 -> [iL]
  Duty_pfc/1 -> Rate Transition/1  "duty"
  Gain2/1 -> Unit Delay2/1
  Unit Delay2/1 -> Simulink-PS Converter1/1
  Rate Transition/1 -> Relational Operator/2
  Data Type Conversion3/1 -> [iout]
  PS-Simulink Converter3/1 -> Data Type Conversion3/1
  [iout] -> Bus Creator/4  "iout"
  Bus Creator/1 -> Sim_feedback/1  "ADC"
  connections:
  Variable Resistor1/LConn2 -- Voltage Sensor/LConn1 -- Capacitor/LConn1 -- Diode9/RConn1
  Voltage Sensor/RConn2 -- Current Sensor1/LConn1 -- Variable Resistor1/RConn1
  Inductor/RConn1 -- Diode9/LConn1 -- "MOSFET (Ideal, Switching)"/RConn1
  Diode1/LConn1 -- Diode7/RConn1 -- Voltage Sensor1/LConn1 -- AC Voltage Source/LConn1
  Diode6/LConn1 -- Diode8/RConn1 -- AC Voltage Source/RConn1 -- Voltage Sensor1/RConn2
  Diode1/RConn1 -- Diode6/RConn1 -- Current Sensor/LConn1
  PS-Simulink Converter2/LConn1 -- Solver Configuration/RConn1 -- Current Sensor/RConn1
  Simulink-PS Converter/RConn1 -- Variable Resistor1/LConn1
  PS-Simulink Converter1/LConn1 -- Voltage Sensor1/RConn1
  PS-Simulink Converter/LConn1 -- Voltage Sensor/RConn1
  Current Sensor/RConn2 -- Inductor/LConn1
  Simulink-PS Converter1/RConn1 -- "MOSFET (Ideal, Switching)"/LConn1
  Diode8/LConn1 -- Capacitor/RConn1 -- Current Sensor1/RConn2 -- Electrical Reference/LConn1 -- "MOSFET (Ideal, Switching)"/RConn2 -- Diode7/LConn1
  PS-Simulink Converter3/LConn1 -- Current Sensor1/RConn1

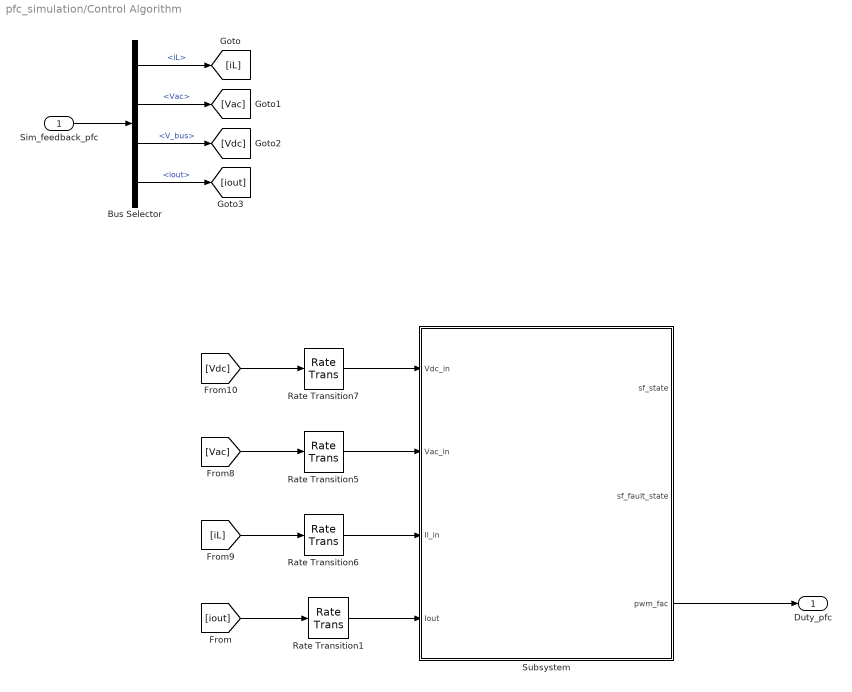
== system pfc_simulation/Control Algorithm ==
  Sim_feedback_pfc : Inport
  Bus Selector : BusSelector  OutputSignals=iL,Vac,V_bus,iout
  Rate Transition{1,5..7} (4 alike) : RateTransition  OutPortSampleTime=Ts
  Subsystem : Subsystem  SystemSampleTime=1/f_sw
  Duty_pfc : Outport
  wires:
  Sim_feedback_pfc/1 -> Bus Selector/1
  [Vac] -> Rate Transition5/1
  Rate Transition5/1 -> Subsystem/2(Vac_in)
  [iL] -> Rate Transition6/1
  Rate Transition6/1 -> Subsystem/3(Il_in)
  Rate Transition7/1 -> Subsystem/1(Vdc_in)
  [Vdc] -> Rate Transition7/1
  Subsystem/3(pwm_fac) -> Duty_pfc/1
  Bus Selector/1 -> [iL]  "<iL>"
  Bus Selector/2 -> [Vac]  "<Vac>"
  Bus Selector/3 -> [Vdc]  "<V_bus>"
  Bus Selector/4 -> [iout]  "<iout>"
  [iout] -> Rate Transition1/1
  Rate Transition1/1 -> Subsystem/4(Iout)

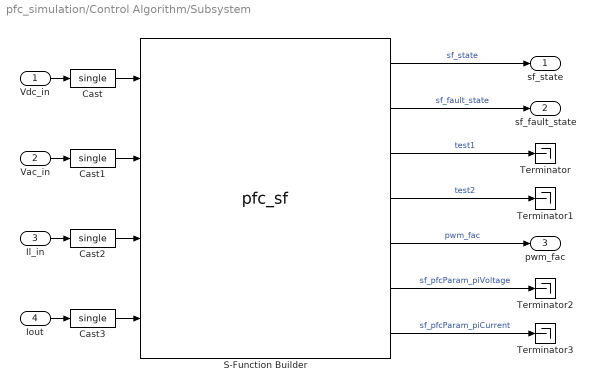
== system pfc_simulation/Control Algorithm/Subsystem ==
  Vdc_in : Inport
  Vac_in : Inport  Port=2
  Il_in : Inport  Port=3
  Iout : Inport  Port=4
  Cast{,1..3} (4 alike) : DataTypeConversion  OutDataTypeStr=single  SaturateOnIntegerOverflow=off  RndMeth=Floor
  S-Function Builder : S-Function  FunctionName=pfc_sf  SFunctionModules=pfc_sf_wrapper.c  SFunctionDeploymentMode=off  EnableBusSupport=off  mask(S-Function Builder){}
      mask help: Simulink:masks:SFunctionBuilder_MD
      mask init:
      | val = [[.9  0.75 0.75 1 1 .9 .9 1]',[1 1 0.75 0.75 .9 .9 1 .9]'];try , sys = get_param(gcb,'SfunBuilderFcnName');if isempty(sys), sys = get_param(gcb,'FunctionName'); end,catch, sys = get_param(gcb,'FunctionName'); end
      settings: CopyFcn=set_param(gcbh,'LinkStatus','none')  OpenFcn=sfunctionwizard(gcbh)
      mask Display:
      | plot(val(:,1),val(:,2))
      | disp(sys)
      | port_label('input',1,sprintf('%s', 'Vdc\_in'),'interpreter','tex')
      | port_label('input',2,sprintf('%s', 'Vac\_in'),'interpreter','tex')
      | port_label('input',3,sprintf('%s', 'Il\_in'),'interpreter','tex')
      | port_label('input',4,sprintf('%s', 'Iout\_in'),'interpreter','tex')
      | port_label('output',1,sprintf('%s', 'state\_out'),'interpreter','tex')
      | port_label('output',2,sprintf('%s', 'fault\_status\_out'),'interpreter','tex')
      | port_label('output',3,sprintf('%s', 'test1'),'interpreter','tex')
      | port_label('output',4,sprintf('%s', 'test2'),'interpreter','tex')
      | port_label('output',5,sprintf('%s', 'pwm\_fac'),'interpreter','tex')
      | port_label('output',6,sprintf('%s', 'pfcParam\_piVoltage\_out'),'interpreter','tex')
      | port_label('output',7,sprintf('%s', 'pfcParam\_piCurrent\_out'),'interpreter','tex')
  Terminator{,1..3} (4 alike) : Terminator
  sf_state : Outport
  sf_fault_state : Outport  Port=2
  pwm_fac : Outport  Port=3
  wires:
  Vdc_in/1 -> Cast/1
  Vac_in/1 -> Cast1/1
  S-Function Builder/4 -> Terminator1/1  "test2"
  S-Function Builder/1 -> sf_state/1  "sf_state"
  S-Function Builder/3 -> Terminator/1  "test1"
  Il_in/1 -> Cast2/1
  S-Function Builder/5 -> pwm_fac/1  "pwm_fac"
  Cast/1 -> S-Function Builder/1
  Cast1/1 -> S-Function Builder/2
  Cast2/1 -> S-Function Builder/3
  S-Function Builder/2 -> sf_fault_state/1  "sf_fault_state"
  S-Function Builder/6 -> Terminator2/1  "sf_pfcParam_piVoltage"
  S-Function Builder/7 -> Terminator3/1  "sf_pfcParam_piCurrent"
  Cast3/1 -> S-Function Builder/4
  Iout/1 -> Cast3/1
